simulink model "stm32f4_basicpwm_demo"  (Simulink 7.3)
settings: Solver=FixedStepDiscrete  SolverMode=SingleTasking  StartTime=0.0  StopTime=10.0  RelTol=1e-3
PreLoadFcn:
  | waijung.modelPreload; % Required for working with Waijung Blockset. Do not remove.
undefined symbols (not defined in the file): HSEOSC, Link, LQFP176, ST, STM32F417IG
libraries: simulink x1, stm32f4_device_config_lib x1
CloseFcn:
  | waijung.modelClose; % Required for working with Waijung Blockset. Do not remove.
settings Model: Creator=Krisada  LastModifiedBy=Krisada
settings OptimizationCC: OptimizeModelRefInitCode=on  LifeSpan=1
settings HardwareCC: ProdEndianess=LittleEndian  ProdHWDeviceType=ARM Compatible->Cortex - M4  TargetEndianess=LittleEndian  TargetHWDeviceType=ARM Compatible->Cortex - M4
settings RTWCC: SystemTargetFile=stm32f4.tlc  GenerateMakefile=off  TemplateMakefile=ert_default_tmf  Description=STM32F4 Target  RetainRTWFile=on  ProcessScript=stm32f4_make_rtw_hook
settings CodeAppCC: IgnoreCustomStorageClasses=off
settings STFCustomTargetCC: ModelReferenceCompliant=off  CombineOutputUpdateFcns=on  ERTCustomFileBanners=on  SupportContinuousTime=off  SupportNonInlinedSFcns=off  SystemTargetFile=stm32f4.tlc
settings ERTTargetCC: MultiwordLength=2048  ModelReferenceCompliant=off  ParMdlRefBuildCompliant=off  CompOptLevelCompliant=off  ERTFirstTimeCompliant=off  ModelStepFunctionPrototypeControlCompliant=off  CPPClassGenCompliant=off  ExtModeMexFile=noextcomm  InlinedParameterPlacement=NonHierarchical  ERTSrcFileBannerTemplate=stm32f4_code_template.cgt  ERTHdrFileBannerTemplate=stm32f4_code_template.cgt  ERTDataSrcFileTemplate=stm32f4_code_template.cgt  ERTDataHdrFileTemplate=stm32f4_code_template.cgt  ERTCustomFileTemplate=stm32f4_file_process.tlc

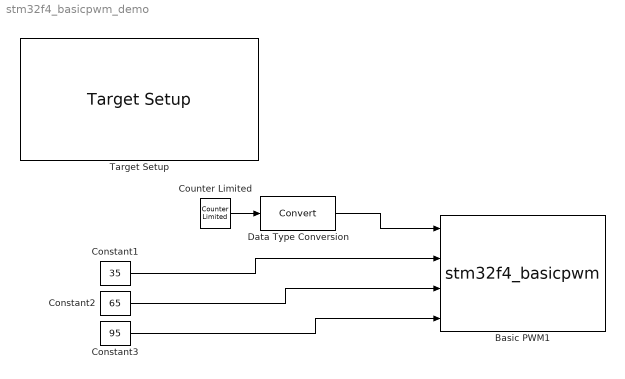
== system stm32f4_basicpwm_demo ==
  Basic PWM1 : S-Function  FunctionName=stm32f4_basicpwm  Parameters=timer,pwmperiod,ch1pin,ch2pin,ch3pin,ch4pin,sampletime,sampletimestr,blockid,apb,portstr,pinstr,pinmat,timarr,timprescale,chmat,polaritystr  EnableBusSupport=off  mask(stm32f4_basicpwm){timer=2, pwmperiod=0.02, polarity=Active High, polaritystr=TIM_OCPolarity_High, ch1pin=A0, ch2pin=A1, ch3pin=A2, ch4pin=B11, sampletime=0.1, sampletimestr=0.1, blockid=BasicPWM1, portpinstr=A0,A1,A2,B11, enablecustomportlabel=off, cinputportlabel=In1, In2, In3, In4, coutputportlabel=0, apb=1, portstr=["A","B"], pinstr=["GPIO_Pin_0 | GPIO_Pin_1 | GPIO_Pin_2","GPIO_Pin_11"], pinmat=[3 0 1 2;1 11 0 0], timarr=64614, timprescale=25, chmat=[1  2  3  4]}
      mask prompts: pwmperiod "PWM Period (seconds)"; ch1pin "Channel 1"; ch2pin "Channel 2"; ch3pin "Channel 3"; ch4pin "Channel 4"; sampletime "Sample time (sec)"; sampletimestr "Compiled sample time (sec) in string"; portpinstr "Port pin string"; enablecustomportlabel "Enable custom port labels"; cinputportlabel "Custom input port labels (Ex. In1, In2, In3)"; coutputportlabel "Custom output port labels (Ex. Out1, Out2, Out3)"; portstr "Port string"; pinstr "Pin string"; pinmat "Pin matrix"; timarr "Timer ARR"; timprescale "Timer PRESCALE"; chmat "Channel order"
      mask help:
      | This block implements basic Edge-aligned Pulse Width Modulation (PWM) generation.
      | All timers are 16-bit. The PWM period is fixed (per timer).
      mask init:
      | stm32f4_basicpwm_callback('init');
      mask Help: web(fullfile(waijungdocroot,'stm32f4_basicpwm.htm'),'-browser')
      mask StyleString: popup(1|2|3|4|5|8|9|10|11|12|13|14),edit,popup(Active High|Active Low),edit,popup(Not available - Do not use|A0|A5|A15),popup(Not available - Do not use|A1|B3),popup(Not available - Do not use|A2|B10),popup(Not available - Do not use|A3|B11),edit,edit,edit,edit,checkbox,edit,edit,edit,edit,edit,edit,edit,edit,edit
      mask CallbackString: stm32f4_basicpwm_callback('timer');|stm32f4_basicpwm_callback('pwmperiod');|stm32f4_basicpwm_callback('polarity');||stm32f4_basicpwm_callback('ch1pin');|stm32f4_basicpwm_callback('ch2pin');|stm32f4_basicpwm_callback('ch3pin');|stm32f4_basicpwm_callback('ch4pin');|stm32f4_basicpwm_callback('sampletime');|stm32f4_basicpwm_callback('sampletimestr');|stm32f4_basicpwm_callback('blockid');||stm32f4_basicpwm_callback('enablecustomportlabel');|||||||||
      mask Display: text(0.95, 0.5, 'Timer: 2\nPolarity: Active High\nPeriod (sec) 0.02\nTs (sec): 0.1','ver','middle','hor','right');port_label('input', 1,'CH1 (A0)');port_label('input', 2,'CH2 (A1)');port_label('input', 3,'CH3 (A2)');port_label('input', 4,'CH4 (B11)')
  Constant1 : Constant  Value=35  OutDataType=fixdt(1, 16)  OutScaling=2^0
  Constant2 : Constant  Value=65  OutDataType=fixdt(1, 16)  OutScaling=2^0
  Constant3 : Constant  Value=95  OutDataType=fixdt(1, 16)  OutScaling=2^0
  Counter Limited : simulink/Sources/Counter Limited  SystemSampleTime=-1  uplimit=20  tsamp=-1
  Data Type Conversion : DataTypeConversion  OutDataType=fixdt(1, 16)  OutScaling=2^0
  Target Setup : stm32f4_device_config_lib/Target Setup  Priority=100  compiler=GNU ARM  previous_compiler=GNU ARM  mcu=STM32F417IG (LQFP176)  mcustr=STM32F417IG  clockconfig=HSEOSC-8MHz  system_stm32f4xx_c_path=F:\trunk\targets\stm32f4_target\stm32f4\utils\system_stm32f4xx_default\STM32F40_41xxx\hseosc8mhz  showmemoryconfiguration=off  stacksize=0x400  heapsize=0x200  enableautocompiledownload=on  fullchiperase=off  programmerinterface=ST-Link  editctrlstr=on  compilercontrolstr=$(patsubst %, -I%, .) -mcpu=cortex-m4 -mthumb -mthumb-interwork -mfloat-abi=hard -mfpu=fpv4-sp-d16 -ffast-math -Wall -Wextra -Ofast  assemblercontrolstr=$(patsubst %, -I%, .) -mcpu=cortex-m4 -mthumb -mthumb-interwork -mfloat-abi=hard -mfpu=fpv4-sp-d16 -ffast-math -Wall -Wextra -Ofast -Wa,-amhls=$(<:.s=.lst) -D__STACK_SIZE=$(STACK_SIZE) -D__HEAP_SIZE=$(HEAP_SIZE)  linkercontrolstr=-T$(LD_SCRIPT) -g -Wl,-Map=$(MAP),--cref,--no-warn-mismatch -mcpu=cortex-m4 -mthumb -mthumb-interwork -mfloat-abi=hard -mfpu=fpv4-sp-d16  runafterdownload=on  execprofile=None  profileruart=3  profilerbaud=115200  profilertxpin=D8  profilerinitstr=0.01,168000000,1680000,115200,0  manualsetsampletime=off  sampletime=0.01  blockid=TargetSetup  systickreloadvalue=1680000  hseval=8000000  lastprofileruart=3  hclk=168000000  flashorigin=0x8000000  flashlength=1024k  ramorigin=0x20000000  ramlength=128k  useextram=off
  wires:
  Counter Limited/1 -> Data Type Conversion/1
  Data Type Conversion/1 -> Basic PWM1/1
  Constant1/1 -> Basic PWM1/2
  Constant2/1 -> Basic PWM1/3
  Constant3/1 -> Basic PWM1/4
